simulink model "Overcurrent_relay"  (R2023b)
settings: Solver=VariableStepAuto  StartTime=0.0  StopTime=10.0  RelTol=1e-3
libraries: spsRMSLib x3, simulink_extras x3
settings Model: Creator=SWARUP  LastModifiedBy=SWARUP

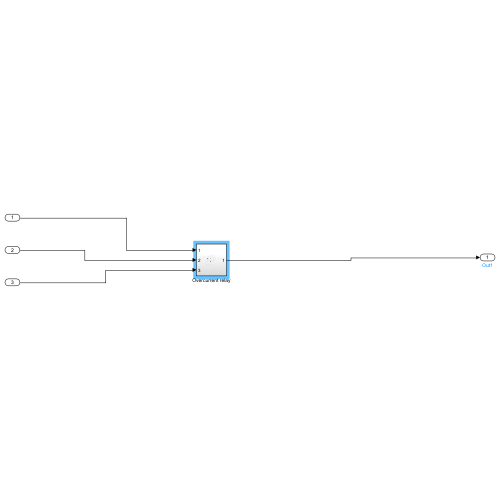
[thumbnail: Simulink's stored preview of the top-level diagram]
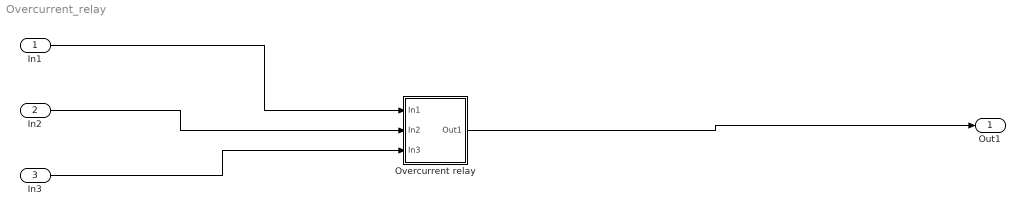
== system Overcurrent_relay ==
  In1 : Inport
  In2 : Inport  Port=2
  In3 : Inport  Port=3
  Overcurrent relay : Subsystem
  Out1 : Outport
  wires:
  In1/1 -> Overcurrent relay/1(In1)
  In2/1 -> Overcurrent relay/2(In2)
  In3/1 -> Overcurrent relay/3(In3)
  Overcurrent relay/1(Out1) -> Out1/1

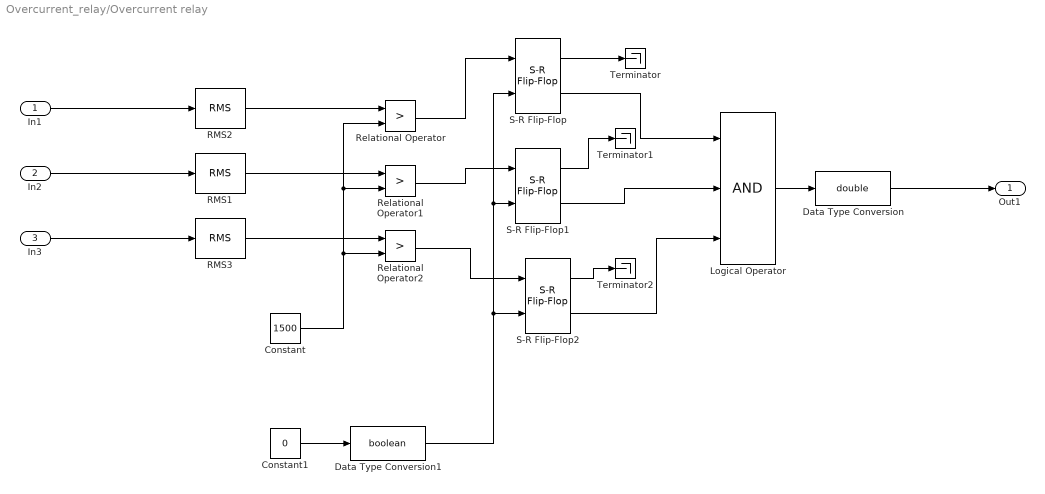
== system Overcurrent_relay/Overcurrent relay ==
  In1 : Inport
  In2 : Inport  Port=2
  In3 : Inport  Port=3
  Constant : Constant  Value=1500
  Constant1 : Constant  Value=0
  Data Type Conversion : DataTypeConversion  OutDataTypeStr=double  SaturateOnIntegerOverflow=off  RndMeth=Floor
  Data Type Conversion1 : DataTypeConversion  OutDataTypeStr=boolean  SaturateOnIntegerOverflow=off  RndMeth=Floor
  Logical Operator : Logic  Inputs=3  AllPortsSameDT=off  OutDataTypeStr=boolean
  RMS1 : spsRMSLib/RMS  TrueRMS=on  Freq=50  RMSInit=0  Ts=0.001
  RMS2 : spsRMSLib/RMS  TrueRMS=on  Freq=50  RMSInit=0  Ts=0.001
  RMS3 : spsRMSLib/RMS  TrueRMS=on  Freq=50  RMSInit=0  Ts=0.001
  Relational Operator : RelationalOperator  Operator=>  OutDataTypeStr=boolean  InputSameDT=off
  Relational Operator1 : RelationalOperator  Operator=>  OutDataTypeStr=boolean  InputSameDT=off
  Relational Operator2 : RelationalOperator  Operator=>  OutDataTypeStr=boolean  InputSameDT=off
  S-R Flip-Flop : simulink_extras/Flip Flops/S-R Flip-Flop  initial_condition=0
  S-R Flip-Flop1 : simulink_extras/Flip Flops/S-R Flip-Flop  initial_condition=0
  S-R Flip-Flop2 : simulink_extras/Flip Flops/S-R Flip-Flop  initial_condition=0
  Terminator : Terminator
  Terminator1 : Terminator
  Terminator2 : Terminator
  Out1 : Outport
  wires:
  Constant/1 -> Relational Operator2/2, Relational Operator1/2, Relational Operator/2
  In3/1 -> RMS3/1
  Relational Operator/1 -> S-R Flip-Flop/1
  RMS1/1 -> Relational Operator1/1
  In1/1 -> RMS2/1
  S-R Flip-Flop1/1 -> Terminator1/1
  S-R Flip-Flop1/2 -> Logical Operator/2
  S-R Flip-Flop2/2 -> Logical Operator/3
  S-R Flip-Flop2/1 -> Terminator2/1
  S-R Flip-Flop/2 -> Logical Operator/1
  RMS2/1 -> Relational Operator/1
  Relational Operator1/1 -> S-R Flip-Flop1/1
  RMS3/1 -> Relational Operator2/1
  Logical Operator/1 -> Data Type Conversion/1
  Data Type Conversion/1 -> Out1/1
  In2/1 -> RMS1/1
  Relational Operator2/1 -> S-R Flip-Flop2/1
  S-R Flip-Flop/1 -> Terminator/1
  Constant1/1 -> Data Type Conversion1/1
  Data Type Conversion1/1 -> S-R Flip-Flop2/2, S-R Flip-Flop1/2, S-R Flip-Flop/2
